simulink model "FSM"  (R2024b)
settings: Solver=FixedStepDiscrete  StartTime=0.0  StopTime=10.0  FixedStep=0.1  RelTol=1e-3  EnableMultiTasking=on
libraries: simulink x8
settings Model: Creator=JuanAntonio  LastModifiedBy=JuanAntonio
settings SolverCC: AlgebraicLoopSolver=TrustRegion  AutoInsertRateTranBlk=on
settings DataIOCC: LimitDataPoints=on
settings OptimizationCC: LifeSpan=inf
settings DebuggingCC: UnconnectedInputMsg=warning  UnconnectedOutputMsg=warning  UnconnectedLineMsg=warning  AllowSymbolicDim=off  SFUnexpectedBacktrackingDiag=warning  SFNoUnconditionalDefaultTransitionDiag=warning  SFOutputUsedAsStateInMooreChartDiag=none  SFExecutionAtInitializationDiag=none  ArithmeticOperatorsInVariantConditions=warning
settings ModelReferenceCC: EnableRefExpFcnMdlSchedulingChecks=on
settings SFSimCC: SimUseLocalCustomCode=off  CustomCodeUndefinedFunction=UseInterfaceOnly
settings RTWCC: RTWUseLocalCustomCode=off  GPUComputeCapability=3.5  DLArmComputeVersion=19.05
settings CodeAppCC: StateflowObjectComments=on
settings GRTTargetCC: TargetLangStandard=C89/C90 (ANSI)
settings ConfigComp: CovMetricSettings=dw  CovSaveCumulativeToWorkspaceVar=on  CovSaveSingleToWorkspaceVar=on  CovExternalEMLEnable=off  CovSFcnEnable=off

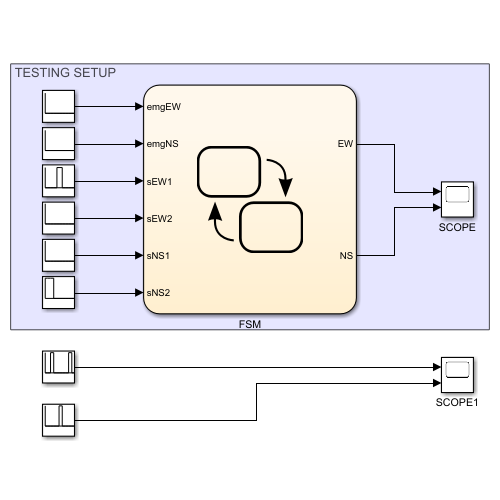
[thumbnail: Simulink's stored preview of the top-level diagram]
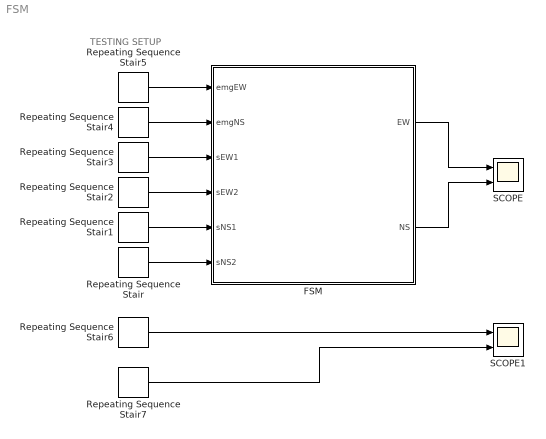
== system FSM ==
  note: TESTING SETUP
  FSM : Stateflow chart  TreatAsAtomicUnit=on
  Repeating Sequence Stair : simulink/Sources/Repeating Sequence Stair  OutValues=[1 1 1 0 0 0 0 0 0 0].'  tsamp=1  OutMin=[]  OutMax=[]  OutDataTypeStr=double  OutputDataTypeScalingMode=double  OutDataType=fixdt(0,8)  ConRadixGroup=Best Precision: Vector-wise  OutScaling=2^-12
  Repeating Sequence Stair{1..2,4..5} (4 alike) : simulink/Sources/Repeating Sequence Stair  OutValues=[0 0 0 0 0 0 0 0 0 0].'  tsamp=1  OutMin=[]  OutMax=[]  OutDataTypeStr=double  OutputDataTypeScalingMode=double  OutDataType=fixdt(0,8)  ConRadixGroup=Best Precision: Vector-wise  OutScaling=2^-12
  Repeating Sequence Stair3 : simulink/Sources/Repeating Sequence Stair  OutValues=[0 0 0 0 1 1 0 0 0 0].'  tsamp=1  OutMin=[]  OutMax=[]  OutDataTypeStr=double  OutputDataTypeScalingMode=double  OutDataType=fixdt(0,8)  ConRadixGroup=Best Precision: Vector-wise  OutScaling=2^-12
  Repeating Sequence Stair6 : simulink/Sources/Repeating Sequence Stair  OutValues=[0 0 1 0 0 0 0 0 1 0].'  tsamp=1  OutMin=[]  OutMax=[]  OutDataTypeStr=double  OutputDataTypeScalingMode=double  OutDataType=fixdt(0,8)  ConRadixGroup=Best Precision: Vector-wise  OutScaling=2^-12
  Repeating Sequence Stair7 : simulink/Sources/Repeating Sequence Stair  OutValues=[0 0 0 0 0 1 0 0 0 0].'  tsamp=1  OutMin=[]  OutMax=[]  OutDataTypeStr=double  OutputDataTypeScalingMode=double  OutDataType=fixdt(0,8)  ConRadixGroup=Best Precision: Vector-wise  OutScaling=2^-12
  SCOPE : Scope  NumInputPorts=2
  SCOPE1 : Scope  NumInputPorts=2
  wires:
  Repeating Sequence Stair/1 -> FSM/6(sNS2)
  FSM/1(EW) -> SCOPE/1
  Repeating Sequence Stair5/1 -> FSM/1(emgEW)
  Repeating Sequence Stair4/1 -> FSM/2(emgNS)
  Repeating Sequence Stair3/1 -> FSM/3(sEW1)
  Repeating Sequence Stair2/1 -> FSM/4(sEW2)
  Repeating Sequence Stair1/1 -> FSM/5(sNS1)
  FSM/2(NS) -> SCOPE/2
  Repeating Sequence Stair6/1 -> SCOPE1/1
  Repeating Sequence Stair7/1 -> SCOPE1/2

== stateflow chart FSM/FSM ==
  state STATIC
    (history)
    state NS_G__EW_R
      NS = 1;
      EW = 0;
    state NS_Y__EW_R
      NS = 0;
      EW = 0;
    state NS_R__EW_R0
      NS = 0;
      EW = 0;
    state NS_R__EW_R1
      NS = 0;
      EW = 0;
    state NS_R__EW_Y
      NS = 0;
      EW = 0;
    state NS_R__EW_G
      NS = 0;
      EW = 1;
    (default) -> STATIC.NS_G__EW_R
    STATIC.NS_R__EW_R1 -> STATIC.NS_G__EW_R [order 2] : [t >= 2]{t = 0}
    STATIC.NS_G__EW_R -> STATIC.NS_Y__EW_R [order 2] : [t >= 8]{t = 0}
    STATIC.NS_Y__EW_R -> STATIC.NS_R__EW_R0 [order 2] : [t >= 2]{t = 0}
    STATIC.NS_R__EW_R0 -> STATIC.NS_R__EW_G [order 2] : [t >= 2]{t = 0}
    STATIC.NS_G__EW_R -> STATIC.NS_G__EW_R [order 1] : [t < 8]{t = t+1}
    STATIC.NS_Y__EW_R -> STATIC.NS_Y__EW_R [order 1] : [t < 2]{t = t+1}
    STATIC.NS_R__EW_R0 -> STATIC.NS_R__EW_R0 [order 1] : [t < 2]{t = t+1}
    STATIC.NS_R__EW_Y -> STATIC.NS_R__EW_Y [order 1] : [t < 2]{t = t+1}
    STATIC.NS_R__EW_G -> STATIC.NS_R__EW_G [order 1] : [t < 8]{t = t+1}
    STATIC.NS_R__EW_R1 -> STATIC.NS_R__EW_R1 [order 1] : [t < 2]{t = t+1}
    STATIC.NS_R__EW_Y -> STATIC.NS_R__EW_R1 [order 2] : [t >= 2]{t = 0}
    STATIC.NS_R__EW_G -> STATIC.NS_R__EW_Y [order 2] : [t >= 8]{t = 0}
  state INIT
  state DYNAMIC
    state NS_G__EW_R
      NS = 1;
      EW = 0;
    state NS_Y__EW_R
      NS = 0;
      EW = 0;
    state NS_R__EW_R0
      NS = 0;
      EW = 0;
    state NS_R__EW_R1
      NS = 0;
      EW = 0;
    state NS_R__EW_Y
      NS = 0;
      EW = 0;
    state NS_R__EW_G
      NS = 0;
      EW = 1;
    (default) -> DYNAMIC.NS_G__EW_R
    DYNAMIC.NS_R__EW_R1 -> DYNAMIC.NS_G__EW_R [order 2] : [t >= 2]{t = 0}
    DYNAMIC.NS_G__EW_R -> DYNAMIC.NS_Y__EW_R [order 2] : [t >= 5 && (sEW1 || sEW2)]{t = 0}
    DYNAMIC.NS_Y__EW_R -> DYNAMIC.NS_R__EW_R0 [order 2] : [t >= 2]{t = 0}
    DYNAMIC.NS_R__EW_R0 -> DYNAMIC.NS_R__EW_G [order 2] : [t >= 2]{t = 0}
    DYNAMIC.NS_G__EW_R -> DYNAMIC.NS_Y__EW_R [order 3] : [t >= 15 && ~(sNS1 || sNS2)]{t = 0}
    DYNAMIC.NS_G__EW_R -> DYNAMIC.NS_G__EW_R [order 1] : [t < 8 || (~sEW1 && ~sEW2)]{t = t+1}
    DYNAMIC.NS_Y__EW_R -> DYNAMIC.NS_Y__EW_R [order 1] : [t < 2]{t = t+1}
    DYNAMIC.NS_R__EW_R0 -> DYNAMIC.NS_R__EW_R0 [order 1] : [t < 2]{t = t+1}
    DYNAMIC.NS_R__EW_R1 -> DYNAMIC.NS_R__EW_R1 [order 1] : [t < 2]{t = t+1}
    DYNAMIC.NS_R__EW_Y -> DYNAMIC.NS_R__EW_Y [order 1] : [t < 2]{t = t+1}
    DYNAMIC.NS_R__EW_G -> DYNAMIC.NS_R__EW_G [order 1] : [t < 8 || (~sNS1 && ~sNS2)]{t = t+1}
    DYNAMIC.NS_R__EW_G -> DYNAMIC.NS_R__EW_Y [order 3] : [t >= 15 && ~(sEW1 || sEW2)]{t = 0}
    DYNAMIC.NS_R__EW_Y -> DYNAMIC.NS_R__EW_R1 [order 2] : [t >= 2]{t = 0}
    DYNAMIC.NS_R__EW_G -> DYNAMIC.NS_R__EW_Y [order 2] : [t >= 8]{t = 0}
  state EMERGENCY
    (history)
    state NS_G__EW_R
      NS = 1;
      EW = 0;
    state NS_Y__EW_R
      NS = 0;
      EW = 0;
    state NS_R__EW_R0
      NS = 0;
      EW = 0;
    state NS_R__EW_R1
      NS = 0;
      EW = 0;
    state NS_R__EW_Y
      NS = 0;
      EW = 0;
    state NS_R__EW_G
      NS = 0;
      EW = 1;
    (default) -> EMERGENCY.NS_G__EW_R
    EMERGENCY.NS_R__EW_R1 -> EMERGENCY.NS_G__EW_R [order 2] : [t >= 2]{t = 0}
    EMERGENCY.NS_G__EW_R -> EMERGENCY.NS_Y__EW_R [order 2] : [~emgNS]{t = 0}
    EMERGENCY.NS_Y__EW_R -> EMERGENCY.NS_R__EW_R0 [order 2] : [t >= 2]{t = 0}
    EMERGENCY.NS_R__EW_R0 -> EMERGENCY.NS_R__EW_G [order 2] : [t >= 2]{t = 0}
    EMERGENCY.NS_G__EW_R -> EMERGENCY.NS_G__EW_R [order 1] : [emgNS]{t = t+1}
    EMERGENCY.NS_Y__EW_R -> EMERGENCY.NS_Y__EW_R [order 1] : [t < 2]{t = t+1}
    EMERGENCY.NS_R__EW_R0 -> EMERGENCY.NS_R__EW_R0 [order 1] : [t < 2]{t = t+1}
    EMERGENCY.NS_R__EW_R1 -> EMERGENCY.NS_R__EW_R1 [order 1] : [t < 2]{t = t+1}
    EMERGENCY.NS_R__EW_Y -> EMERGENCY.NS_R__EW_Y [order 1] : [t < 2]{t = t+1}
    EMERGENCY.NS_R__EW_G -> EMERGENCY.NS_R__EW_G [order 1] : [emgEW]{t = t+1}
    EMERGENCY.NS_R__EW_Y -> EMERGENCY.NS_R__EW_R1 [order 2] : [t >= 2]{t = 0}
    EMERGENCY.NS_R__EW_G -> EMERGENCY.NS_R__EW_Y [order 2] : [~emgEW]{t = 0}
  (default) -> INIT
  INIT -> STATIC : {t = 0}
  EMERGENCY -> STATIC [order 2] : [~emgNS && ~emgEW && ~((sNS1 || sNS2) && (sEW1 || sEW2))]
  STATIC -> EMERGENCY [order 2] : [emgNS || emgEW]
  DYNAMIC -> STATIC [order 2] : [((sNS1 || sNS2) && (sEW1 || sEW2))]
  STATIC -> DYNAMIC [order 1] : [~((sNS1 || sNS2) && (sEW1 || sEW2))]
  EMERGENCY -> DYNAMIC [order 1] : [~emgNS && ~emgEW && ~((sNS1 || sNS2) && (sEW1 || sEW2))]
  DYNAMIC -> EMERGENCY [order 1] : [emgNS || emgEW]
  data: EW output; NS output; t local; emgEW input; emgNS input; sEW1 input; sEW2 input; sNS1 input; sNS2 input
